simulink model "autosar_bsw_inject_test"  (R2022b)
settings: Solver=VariableStepAuto  StartTime=0.0  StopTime=Inf  RelTol=1e-3  EnableMultiTasking=on
libraries: autosarlibdem x2
settings Model: PacingRate=2  Creator=The MathWorks, Inc.  LastModifiedBy=The MathWorks, Inc.
settings SolverCC: AutoInsertRateTranBlk=on  MaxZcPerStep=1
settings OptimizationCC: DefaultParameterBehavior=Inlined  EnhancedBackFolding=on  PassReuseOutputArgsAs=Individual arguments  ZeroExternalMemoryAtStartup=off  ZeroInternalMemoryAtStartup=off  OptimizeBlockOrder=speed  DifferentSizesBufferReuse=on  OptimizationCustomize=off  EfficientTunableParamExpr=on
settings DebuggingCC: ParameterTunabilityLossMsg=error
settings ModelReferenceCC: EnableRefExpFcnMdlSchedulingChecks=on
settings SFSimCC: MATLABDynamicMemAlloc=off
settings RTWCC: Description=AUTOSAR  SystemTargetFile=autosar.tlc  GenCodeOnly=on  TemplateMakefile=ert_default_tmf  DLArmComputeVersion=19.05
settings CodeAppCC: ForceParamTrailComments=on  IgnoreCustomStorageClasses=off  OperatorAnnotations=on  SimulinkDataObjDesc=on  SFDataObjDesc=on  InsertBlockDesc=on
settings STFCustomTargetCC: TargetLangStandard=C99 (ISO)  MultiwordLength=256  ParMdlRefBuildCompliant=on  CompOptLevelCompliant=on  IncludeMdlTerminateFcn=off  CombineOutputUpdateFcns=on  SuppressErrorStatus=on  ERTCustomFileBanners=on  SupportNonFinite=off  SupportComplex=off  SupportContinuousTime=off  SupportNonInlinedSFcns=off  RemoveResetFunc=on  MATLABClassNameForMDSCustomization=Simulink.SoftwareTarget.ERTCustomization  AutosarCompliant=on  UseToolchainInfoCompliant=on  LookupTableObjectStructAxisOrder=2,1,3,4,...  LUTObjectStructOrderEvenSpacing=Size,Table,Breakpoints  SystemTargetFile=autosar.tlc
settings ERTTargetCC: TargetLangStandard=C99 (ISO)  ConcurrentExecutionCompliant=off  IncludeMdlTerminateFcn=off  SuppressErrorStatus=on  SupportNonFinite=off  SupportComplex=off  ModelStepFunctionPrototypeControlCompliant=off  CPPClassGenCompliant=off  AutosarCompliant=on  LookupTableObjectStructAxisOrder=2,1,3,4,...  LUTObjectStructOrderEvenSpacing=Size,Table,Breakpoints  InlinedParameterPlacement=NonHierarchical  ERTCustomFileTemplate=example_file_process.tlc

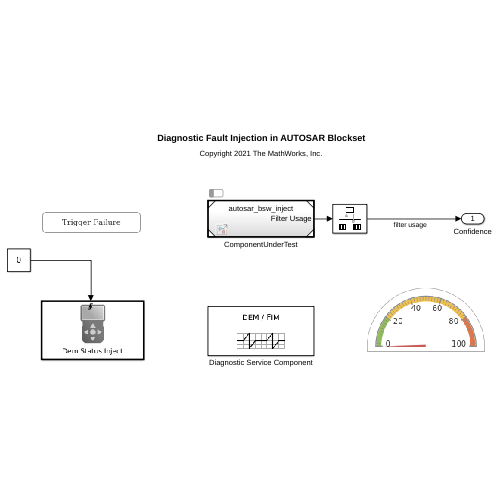
[thumbnail: Simulink's stored preview of the top-level diagram]
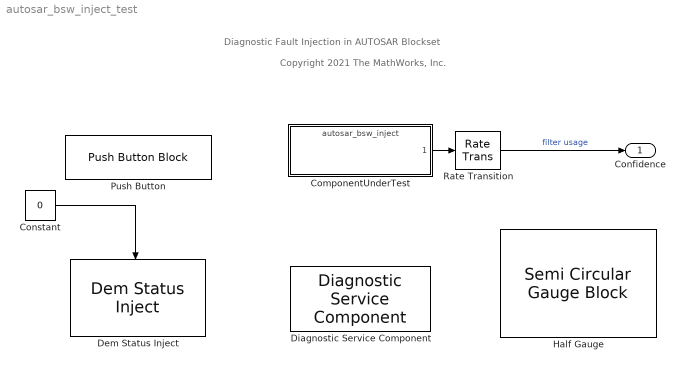
== system autosar_bsw_inject_test ==
  note: Copyright 2021 The MathWorks, Inc.
  note: Diagnostic Fault Injection in AUTOSAR Blockset
  ComponentUnderTest : ModelReference  ModelNameDialog=autosar_bsw_inject  SimulationMode=Normal  ScheduleRates=on  ScheduleRatesWith=Schedule Editor  ModelReferenceVersion=2.0
  Constant : Constant  Value=0
  Dem Status Inject : autosarlibdem/Dem Status Inject  Priority=1  EventId=1  FaultType=Event Fail  TriggerType=rising  InjectTriggerType=rising
  Diagnostic Service Component : autosarlibdem/Diagnostic Service Component  ClientPortNames={'FilterInfo', 'FilterMonitor'}  ClientPortPortDefinedArguments={'1', '1'}  MaxEventId=10  MaxFID=10  DemDebounceCounterIncrementStepSize=1  DemDebounceCounterDecrementStepSize=1  DemDebounceCounterFailedThreshold=2  DemDebounceCounterPassedThreshold=-1  InhibitionMatrix=[0 0 0 0 0 0 0 0 0 0 0;0 0 0 0 0 0 0 0 0 0 0;0 0 0 0 0 0 0 0 0 0 0;0 0 0 0 0 0 0 0 0 0 0;0 0 0 0 0 0 0 0 0 0 0;0 0 0 0 0 0 0 0 0 0 0;0 0 0 0 0 0 0 0 0 0 0;0 0 0 0 0 0 0 0 0 0 0;0 0 0 0 0 0 0 0 0 0 0;0 0 0 0 0 0 0 0 0 0 0;0 0 0 0 0 0 0 0 0 0 0]  EnableConditionIndexes=zeros(257,'uint8')  StorageConditionIndexes=zeros(257,'uint8')
  Half Gauge : SemiCircularGaugeBlock  LabelPosition=Hide
  Push Button : PushButtonBlock  ButtonText=Trigger Failure  OffValue=0.000000
  Rate Transition : RateTransition
  Confidence : Outport
  wires:
  ComponentUnderTest/1 -> Rate Transition/1
  Constant/1 -> Dem Status Inject/Trigger
  Rate Transition/1 -> Confidence/1  "filter usage"
